simulink model "sampleModel136"  (R2021b)
settings: Solver=VariableStepAuto  StartTime=0.0  StopTime=10.0  RelTol=1e-3
undefined symbols (not defined in the file or in its folder): Newton, Raphson
libraries: simulink x3
settings Model: Creator=user  LastModifiedBy=user

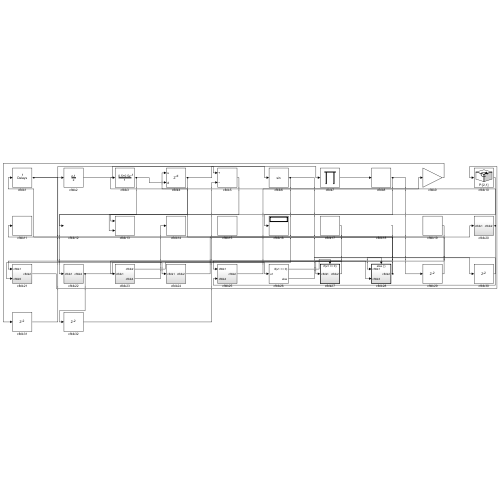
[thumbnail: Simulink's stored preview of the top-level diagram]
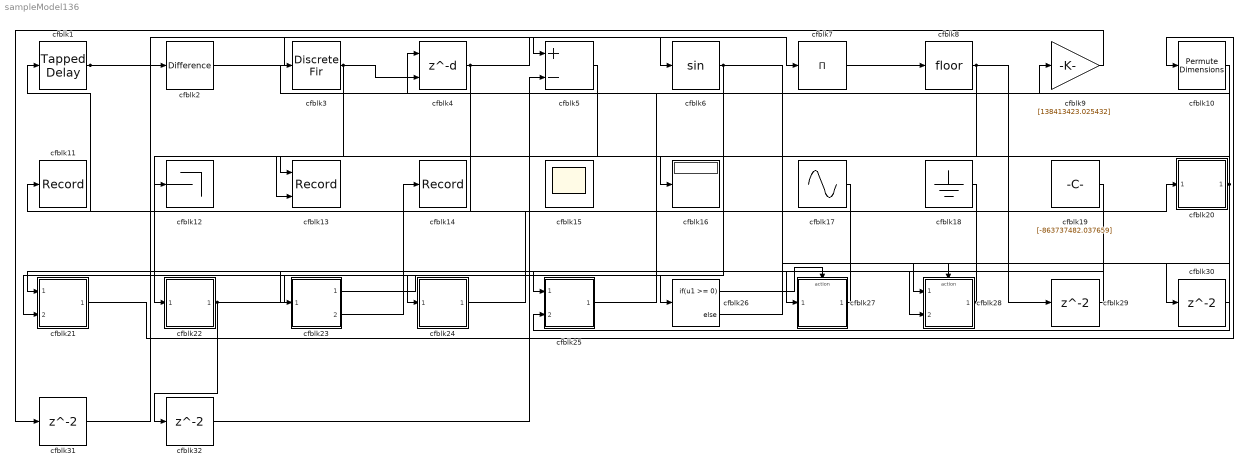
== system sampleModel136 ==
  cfblk1 : simulink/Discrete/Tapped Delay  vinit=0.0  samptime=-1  NumDelays=1  DelayOrder=Oldest  includeCurrent=off
  cfblk10 : PermuteDimensions
  cfblk11 : Record  FileSettingsInternal="{\"entries\":[{\"content\":{\"excelSettings\":{\"content\":{},\"type\":\"Streamout.ExcelSettings\"}},\"type\":\"Streamout.FileSettingStorage\",\"uuid\":\"e239c649-e162-45b1-99e0-f70ca900fe27\"}],\"packageUris\":[\"http://schema.mathworks.com/mf0/streamout_blocks/R2020a\"],\"version\":\"1.0\"}"  SignalsInternal="{\"entries\":[{\"content\":{\"signals\":[{\"content\":{\"blockPath\":[\"sampleModel136/cfblk11\"],\"channel\":[],\"dimensions\":[1],\"domain\":\"sampleModel136/cfblk11\",\"lineColor\":\"#fe330a\",\"plots\":[1],\"port\":1,\"sid\":[\"\"],\"signalID\":4775,\"signalName\":\"cfblk28\"},\"type\":\"RecordBlkView.Signal\",\"uuid\":\"98577bf9-6dcc-42ea-89ac-f543c9a0b2c8\"}]},\"type\":\"RecordBlkView.InputSignals\",\"uuid\":\"1309dedc-c4ce-41f5-a313-656a11216a91\"}],\"packageUris\":[\"http://schema.mathworks.com/mf0/streamout_blocks/R2020a\"],\"version\":\"1.0\"}"  VisualizationBindings="{\"sparklinesplugin\":{\"info\":[{\"bindingParametersList\":[],\"subplotID\":1}]}}"
  cfblk12 : Terminator
  cfblk13 : Record  FileSettingsInternal="{\"entries\":[{\"content\":{\"excelSettings\":{\"content\":{},\"type\":\"Streamout.ExcelSettings\"}},\"type\":\"Streamout.FileSettingStorage\",\"uuid\":\"7e438cff-e1e9-42c2-9201-376bcc0859c7\"}],\"packageUris\":[\"http://schema.mathworks.com/mf0/streamout_blocks/R2020a\"],\"version\":\"1.0\"}"  Layout=[1 1]  SignalsInternal="{\"entries\":[{\"content\":{\"signals\":[{\"content\":{\"blockPath\":[\"sampleModel136/cfblk13\"],\"channel\":[],\"dimensions\":[1],\"domain\":\"sampleModel136/cfblk13\",\"lineColor\":\"#a2142f\",\"plots\":[1],\"port\":1,\"sid\":[\"\"],\"signalID\":4779,\"signalName\":\"cfblk4\"},\"type\":\"RecordBlkView.Signal\",\"uuid\":\"cf575757-36e5-4343-89ff-bcf67058d461\"},{\"content\":{\"blockPath\":[\"sampleModel136/cfblk13\"],\"channel\":[],\"dimensions\":[1],\"domain\":\"sampleModel136/cfblk13\",\"lineColor\":\"#139fff\",\"plots\":[1],\"port\":2,\"sid\":[\"\"],\"signalID\":4783,\"signalName\":\"cfblk3\"},\"type\":\"RecordBlkView.Signal\",\"uuid\":\"a48f6166-5eb8-492e-86f5-e15acc915563\"}]},\"type\":\"RecordBlkView.InputSignals\",\"uuid\":\"fafe21f8-5d1d-494e-b34c-5121a032ddb5\"}],\"packageUris\":[\"http://schema.mathworks.com/mf0/streamout_blocks/R2020a\"],\"version\":\"1.0\"}"  VisualizationBindings="{\"xyplotplugin\":{\"info\":[{\"series\":[{\"bindingParametersList\":[{\"parameter\":\"X-Axis\",\"signalID\":4779,\"signalName\":\"cfblk4\"},{\"parameter\":\"Y-Axis\",\"signalID\":4783,\"signalName\":\"cfblk3\"}],\"seriesID\":50209}],\"subplotID\":1}]}}"  CompatibilityTag=XY
  cfblk14 : Record  FileSettingsInternal="{\"entries\":[{\"content\":{\"excelSettings\":{\"content\":{},\"type\":\"Streamout.ExcelSettings\"}},\"type\":\"Streamout.FileSettingStorage\",\"uuid\":\"a66961b6-6b32-4e46-aeb1-523b8202ddf9\"}],\"packageUris\":[\"http://schema.mathworks.com/mf0/streamout_blocks/R2020a\"],\"version\":\"1.0\"}"  SignalsInternal="{\"entries\":[{\"content\":{\"signals\":[{\"content\":{\"blockPath\":[\"sampleModel136/cfblk14\"],\"channel\":[],\"dimensions\":[1],\"domain\":\"sampleModel136/cfblk14\",\"lineColor\":\"#d95319\",\"plots\":[1],\"port\":1,\"sid\":[\"\"],\"signalID\":4787,\"signalName\":\"cfblk23:2\"},\"type\":\"RecordBlkView.Signal\",\"uuid\":\"cb300982-8b9f-44cb-86a1-47a6627cf367\"}]},\"type\":\"RecordBlkView.InputSignals\",\"uuid\":\"16d4de59-5a7e-4e6e-983c-ef62e5344898\"}],\"packageUris\":[\"http://schema.mathworks.com/mf0/streamout_blocks/R2020a\"],\"version\":\"1.0\"}"  VisualizationBindings="{\"sparklinesplugin\":{\"info\":[{\"bindingParametersList\":[],\"subplotID\":1}]}}"
  cfblk15 : Scope
      settings: Floating=on
  cfblk16 : Display
  cfblk17 : Sin  Amplitude=[-373981479.993645]  Bias=[-414069447.787755]  SampleTime=0
  cfblk18 : Ground
  cfblk19 : Constant  Value=[-863737482.037659]  SampleTime=1
  cfblk2 : simulink/Discrete/Difference  ICPrevInput=0.0  OutMin=[]  OutMax=[]  OutDataTypeStr=Inherit: Inherit via back propagation  OutDataType=fixdt(1, 16)  OutScaling=2^-10  DoSatur=off
  cfblk20 : Subsystem
  cfblk21 : Subsystem
  cfblk22 : Subsystem
  cfblk23 : Subsystem
  cfblk24 : Subsystem
  cfblk25 : Subsystem
  cfblk26 : If  IfExpression=u1 >= 0  SampleTime=1
  cfblk27 : Subsystem  TreatAsAtomicUnit=on
  cfblk28 : Subsystem  TreatAsAtomicUnit=on
  cfblk{29..32} (4 alike) : Delay  SampleTime=1
  cfblk3 : DiscreteFir  SampleTime=1
  cfblk4 : Delay  DelayLengthSource=Input port  SampleTime=1
      settings: InputPortMap=u0,p1
  cfblk5 : Sum  Inputs=+-
  cfblk6 : Trigonometry
  cfblk7 : Product  Inputs=*
  cfblk8 : Rounding
  cfblk9 : Gain  Gain=[138413423.025432]
  wires:
  cfblk27/1(cfblk2) -> cfblk25/1(cfblk1)
  cfblk24/1(cfblk2) -> cfblk20/1(cfblk1)
  cfblk5/1 -> cfblk22/1(cfblk1)
  cfblk6/1 -> cfblk21/2(cfblk5), cfblk30/1
  cfblk7/1 -> cfblk8/1
  cfblk1/1 -> cfblk7/1, cfblk28/2(cfblk3)
  cfblk8/1 -> cfblk12/1, cfblk29/1
  cfblk22/1(cfblk2) -> cfblk24/1(cfblk1), cfblk32/1
  cfblk20/1(cfblk2) -> cfblk25/2(cfblk4), cfblk3/1
  cfblk19/1 -> cfblk27/1(cfblk1)
  cfblk18/1 -> cfblk23/1(cfblk1)
  cfblk23/1(cfblk2) -> cfblk26/1
  cfblk10/1 -> cfblk16/1
  cfblk4/1 -> cfblk13/1, cfblk6/1
  cfblk3/1 -> cfblk13/2, cfblk4/2
  cfblk2/1 -> cfblk5/1
  cfblk25/1(cfblk2) -> cfblk9/1
  cfblk17/1 -> cfblk21/1(cfblk1)
  cfblk23/2(cfblk4) -> cfblk14/1
  cfblk21/1(cfblk2) -> cfblk10/1
  cfblk28/1(cfblk2) -> cfblk4/1, cfblk11/1
  cfblk26/1 -> cfblk27/Action
  cfblk26/2 -> cfblk28/Action
  cfblk29/1 -> cfblk1/1
  cfblk30/1 -> cfblk28/1(cfblk1)
  cfblk9/1 -> cfblk31/1
  cfblk31/1 -> cfblk2/1
  cfblk32/1 -> cfblk5/2

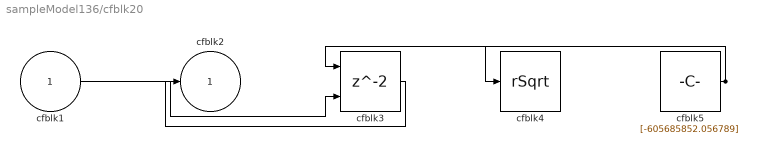
== system sampleModel136/cfblk20 ==
  cfblk1 : Inport
  cfblk3 : Delay  ShowEnablePort=on  SampleTime=1
      settings: InputPortMap=u0,e6
  cfblk4 : Sqrt  Operator=rSqrt  AlgorithmType=Newton-Raphson  SaturateOnIntegerOverflow=on
  cfblk5 : Constant  Value=[-605685852.056789]  SampleTime=1
  cfblk2 : Outport
  wires:
  cfblk5/1 -> cfblk3/1, cfblk4/1
  cfblk1/1 -> cfblk3/2
  cfblk3/1 -> cfblk2/1

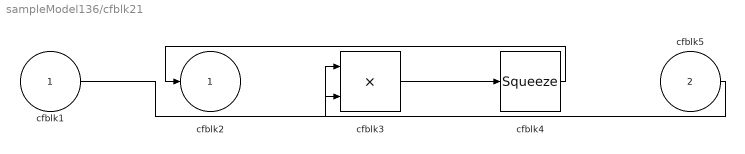
== system sampleModel136/cfblk21 ==
  cfblk1 : Inport
  cfblk5 : Inport  Port=2
  cfblk3 : Product
  cfblk4 : Squeeze
  cfblk2 : Outport
  wires:
  cfblk3/1 -> cfblk4/1
  cfblk4/1 -> cfblk2/1
  cfblk1/1 -> cfblk3/1
  cfblk5/1 -> cfblk3/2

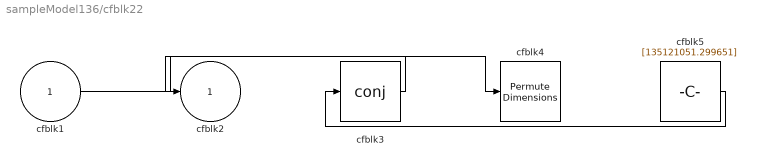
== system sampleModel136/cfblk22 ==
  cfblk1 : Inport
  cfblk3 : Math  Operator=conj  SaturateOnIntegerOverflow=on
  cfblk4 : PermuteDimensions
  cfblk5 : Constant  Value=[135121051.299651]  SampleTime=1
  cfblk2 : Outport
  wires:
  cfblk1/1 -> cfblk4/1
  cfblk5/1 -> cfblk3/1
  cfblk3/1 -> cfblk2/1

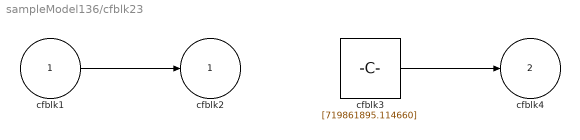
== system sampleModel136/cfblk23 ==
  cfblk1 : Inport
  cfblk3 : Constant  Value=[719861895.114660]  SampleTime=1
  cfblk2 : Outport
  cfblk4 : Outport  Port=2
  wires:
  cfblk3/1 -> cfblk4/1
  cfblk1/1 -> cfblk2/1

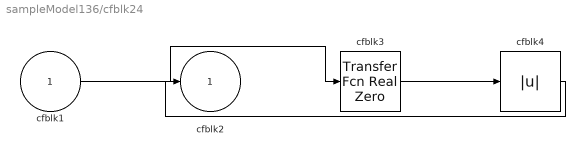
== system sampleModel136/cfblk24 ==
  cfblk1 : Inport
  cfblk3 : simulink/Discrete/Transfer Fcn Real Zero  ZeroZ=0.75  ICPrevInput=0.0  DoSatur=off
      settings: SourceProductBaseCode=SL
  cfblk4 : Abs
  cfblk2 : Outport
  wires:
  cfblk3/1 -> cfblk4/1
  cfblk1/1 -> cfblk3/1
  cfblk4/1 -> cfblk2/1

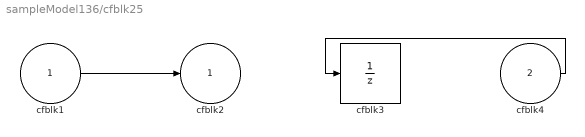
== system sampleModel136/cfblk25 ==
  cfblk1 : Inport
  cfblk4 : Inport  Port=2
  cfblk3 : UnitDelay  HasFrameUpgradeWarning=on
  cfblk2 : Outport
  wires:
  cfblk1/1 -> cfblk2/1
  cfblk4/1 -> cfblk3/1

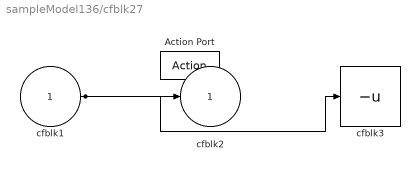
== system sampleModel136/cfblk27 ==
  cfblk1 : Inport
  Action Port : ActionPort  ActionPortLabel=if(u1 >= 0)
  cfblk3 : UnaryMinus
  cfblk2 : Outport
  wires:
  cfblk1/1 -> cfblk2/1, cfblk3/1

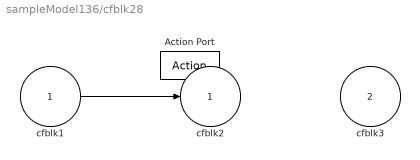
== system sampleModel136/cfblk28 ==
  cfblk1 : Inport
  cfblk3 : Inport  Port=2
  Action Port : ActionPort  ActionPortLabel=else
  cfblk2 : Outport
  wires:
  cfblk1/1 -> cfblk2/1
